simulink model "Transimpedance"  (R2020b)
settings: Solver=VariableStepAuto  StartTime=0.0  StopTime=1  RelTol=1e-3
libraries: fl_lib x7, nesl_utility x3, ee_lib x2
settings Model: Creator=Miodrag Bolic  LastModifiedBy=bolic

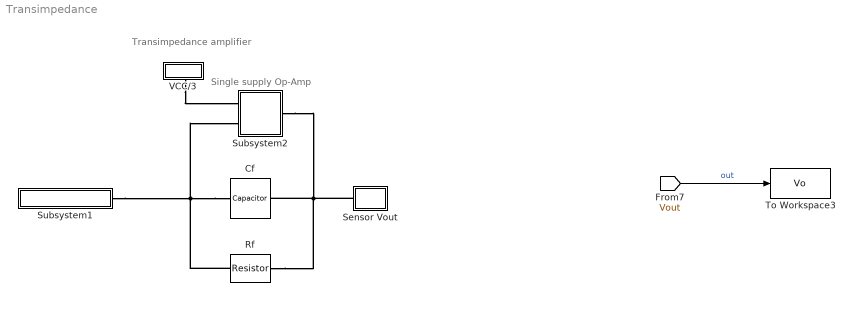
== system Transimpedance ==
  note: Single supply Op-Amp
  note: Transimpedance amplifier
  Cf : fl_lib/Electrical/Electrical Elements/Capacitor  c=2.70 nF  r=0 Ohm  g=0 1/Ohm  i_specify=off  i_priority=High  i=0 A  i_nominal_specify=off  i_nominal_unit=A  i_nominal_value=1  v_specify=off  v_priority=High  v=0 V  v_nominal_specify=off  v_nominal_unit=V  v_nominal_value=1  vc_specify=off  vc_priority=High  vc=0 V  vc_nominal_specify=off  vc_nominal_unit=V  vc_nominal_value=1
      settings: AttributesFormatString=%<c> %<c_unit>  SourceProductName=Foundation Library
  Rf : fl_lib/Electrical/Electrical Elements/Resistor  R=200 kOhm  i_specify=off  i_priority=High  i=0 A  i_nominal_specify=off  i_nominal_unit=A  i_nominal_value=1  v_specify=off  v_priority=High  v=0 V  v_nominal_specify=off  v_nominal_unit=V  v_nominal_value=1
      settings: AttributesFormatString=%<R> %<R_unit>  SourceProductName=Foundation Library
  Sensor Vout : Subsystem
      mask Display: disp('Vo')
  Subsystem1 : Subsystem
      mask Display: disp("Photodetector")
  Subsystem2 : Subsystem
      mask Display: image('op_amp_plus_up.png')
  To Workspace3 : ToWorkspace  VariableName=Vo  SaveFormat=Timeseries  SampleTime=0.001
  VCC/3 : Subsystem
      settings: PortSchema="{\"entries\":[{\"content\":{\"sides\":[{\"content\":{\"connectorIds\":[]},\"type\":\"ConnectorPlacement.EquallySpacedRectSide\",\"uuid\":\"ad0d720a-99c9-4023-9136-2a4b865f3a0c\"},{\"content\":{\"connectorIds\":[],\"side\":\"RIGHT\"},\"type\":\"ConnectorPlacement.EquallySpacedRectSide\",\"uuid\":\"1bfb0966-097c-42b2-b98f-8d518b37dee9\"},{\"content\":{\"connectorIds\":[],\"side\":\"TOP\"},\"type\":\"ConnectorPlacement.EquallySpacedRectSide\",\"uuid\":\"cec6aa57-011f-45b6-ab10-0fe0acad4f73\"},{\"content\":{\"connectorIds\":[\"RConn1\"],\"side\":\"BOTTOM\"},\"type\":\"ConnectorPlacement.EquallySpacedRectSide\",\"uuid\":\"cda8d0ca-8f7a-4c71-b373-22a3b7ce2625\"},{\"content\":{\"connectorIds\":[],\"side\":\"HIDDEN\"},\"type\":\"ConnectorPlacement.EquallySpacedRectSide\",\"uuid\":\"d4614205-975b-463c-8926-95474d0bf73b\"}]},\"type\":\"ConnectorPlacement.EquallySpacedConnector\",\"uuid\":\"1907b430-f891-4093-9422-d2389a8bd2eb\"}],\"packageUris\":[\"http://schema.mathworks.com/mf0/Connector/R2020b\"],\"version\":\"1.0\"}"
      mask Display: disp("Offset")
  wires:
  [Vout] -> To Workspace3/1  "out"
  connections:
  Sensor Vout/LConn1 -- Cf/RConn1 -- Subsystem2/RConn1 -- Rf/RConn1
  VCC/3/RConn1 -- Subsystem2/LConn1
  Cf/LConn1 -- Subsystem2/LConn2 -- Rf/LConn1 -- Subsystem1/RConn1

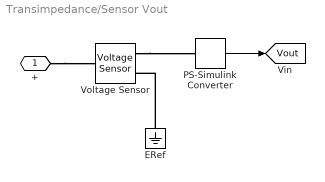
== system Transimpedance/Sensor Vout ==
  ERef : fl_lib/Electrical/Electrical Elements/Electrical Reference
      settings: SourceProductName=Foundation Library
  PS-Simulink Converter : nesl_utility/PS-Simulink Converter  PhysicalDomain=network_engine_domain  SubClassName=ps_output  LeftPortType=input  RightPortType=output  PseudoPeriodic=off  Frequencies=[]  Unit=1  AffineConversion=off
      settings: SourceProductName=Utilities
  Voltage Sensor : fl_lib/Electrical/Electrical Sensors/Voltage Sensor
      settings: SourceProductName=Foundation Library
  + : PMIOPort  Side=Left
  tag scope: Vout=global
  wires:
  PS-Simulink Converter/1 -> [Vout]
  connections:
  ERef/LConn1 -- Voltage Sensor/RConn2
  Voltage Sensor/RConn1 -- PS-Simulink Converter/LConn1
  +/RConn1 -- Voltage Sensor/LConn1

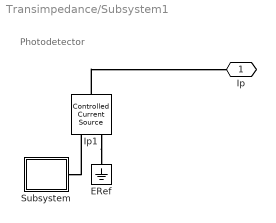
== system Transimpedance/Subsystem1 ==
  note: Photodetector
  ERef : fl_lib/Electrical/Electrical Elements/Electrical Reference
      settings: SourceProductName=Foundation Library
  Ip1 : fl_lib/Electrical/Electrical Sources/Controlled Current Source
  Subsystem : Subsystem
      mask Display: disp("In")
  Ip : PMIOPort  Side=Right
  connections:
  Subsystem/RConn1 -- Ip1/RConn1
  Ip1/RConn2 -- ERef/LConn1
  Ip1/LConn1 -- Ip/RConn1

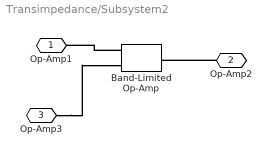
== system Transimpedance/Subsystem2 ==
  Band-Limited Op-Amp : ee_lib/Integrated Circuits/Band-Limited Op-Amp  A=10000  Rin=1e8 Ohm  Rout=100 Ohm  Vmin=0 V  Vmax=3.3 V  Vdotmax=1000 V/s  f=1e6 Hz  V0=0 V
      settings: SourceProductBaseCode=SN
  Op-Amp1 : PMIOPort  Side=Left
  Op-Amp2 : PMIOPort  Port=2  Side=Right
  Op-Amp3 : PMIOPort  Port=3  Side=Left
  connections:
  Band-Limited Op-Amp/LConn1 -- Op-Amp1/RConn1
  Op-Amp3/RConn1 -- Band-Limited Op-Amp/LConn2
  Op-Amp2/RConn1 -- Band-Limited Op-Amp/RConn1

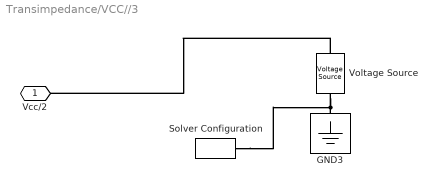
== system Transimpedance/VCC//3 ==
  GND3 : fl_lib/Electrical/Electrical Elements/Electrical Reference
  Solver Configuration : nesl_utility/Solver Configuration  PhysicalDomain=network_engine_domain  SubClassName=solver  LeftPortType=input  RightPortType=generic  Tones=[]  Harmonics=[]  SimulateNoise=off  Profile=off  UseLocalSampling=off  EnableSwitchedLinearOptims=on  FrequencyDomain=off  UseCCode=off  RelTol=0.001  AbsTol=1e-06  MinStep=1e-09  ToWorkspace=off  RevertToSquareIcSolve=off  NumHomotopyIterations=100  PhasorMode=off  PhasorModeNumHarmonics=1  DoDC=off  ResidualTolerance=1e-9  UseLocalSolver=off  LocalSolverChoice=NE_BACKWARD_EULER_ADVANCER  LocalSolverSampleTime=.001  DoFixedCost=off  MaxNonlinIter=3  MaxModeIter=2  ComputeImpulses=off  ImpulseIterations=2  LinearAlgebra=auto  EquationFormulation=NE_TIME_EF  DelaysMemoryBudget=1024  AutomaticFiltering=on  FilteringTimeConstant=0.001  PartitionStorageMethod=AS_NEEDED  PartitionMemoryBudget=1024  PartitionMethod=FAST
  Voltage Source : ee_lib/Sources/Voltage Source  dc_voltage=0.2 V  ac_voltage=0 V  ac_shift=0 rad  ac_frequency=0 Hz  noise_mode=0  PSD=0 V^2/Hz  repeatability=1  auto_seed=2984266212  user_seed=0  sample_time=1e-3 s  i_specify=off  i_priority=None  i=0 A  i_nominal_specify=off  i_nominal_unit=A  i_nominal_value=1  v_specify=off  v_priority=None  v=0 V  v_nominal_specify=off  v_nominal_unit=V  v_nominal_value=1
  "Vcc/2 " : PMIOPort  Side=Right
  connections:
  GND3/LConn1 -- Solver Configuration/RConn1 -- Voltage Source/RConn1
  Voltage Source/LConn1 -- "Vcc/2 "/RConn1

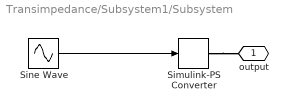
== system Transimpedance/Subsystem1/Subsystem ==
  Simulink-PS Converter : nesl_utility/Simulink-PS Converter  PhysicalDomain=network_engine_domain  SubClassName=ps_input  LeftPortType=input  RightPortType=output  PseudoPeriodic=off  Frequencies=[]  NoiseDistribution=none  NoiseParameters=[]  Unit=1  AffineConversion=off  FilteringAndDerivatives=provide  SimscapeFilterOrder=1  InputFilterTimeConstant=0.001  UdotUserProvided=0
  Sine Wave : Sin  SineType=Sample based  Amplitude=-1e-6  Bias=-1e-6  Samples=500  SampleTime=0.0001
  output : PMIOPort  Side=Right
  wires:
  Sine Wave/1 -> Simulink-PS Converter/1
  connections:
  Simulink-PS Converter/RConn1 -- output/RConn1
